simulink model "sistema_completo_discretizado_final"  (R2023b)
settings: Solver=FixedStepDiscrete  StartTime=0.0  StopTime=10.0  FixedStep=100e-6  RelTol=1e-3
values from neighbouring files (symbols this model uses):
  alpha_Cu = 3.9e-3    (= 0.0039)    [controlador_foc_simulink.m]    (also in parametros_planta.m; params_subsistema_termico.m; sistema_completo_en_codigo.m)
  beq_nom = bm + bl_nom/r^2    (= 2.19444444444e-05)    [parametros_planta.m]    (also in params_subsistema_mecanico.m; sistema_completo_en_codigo.m)
  Cts = 0.818    [parametros_planta.m]    (also in params_subsistema_termico.m)
  Jeq_nom = Jm + Jl_nom/r^2    (= 1.97847222222e-05)    [params_subsistema_mecanico.m]    (also in sistema_completo_en_codigo.m)
  kg_eq_nom = g*kl_nom/r    (= 0.0204305208333)    [params_subsistema_mecanico.m]    (also in sistema_completo_en_codigo.m)
  L_d = 6.6e-3    (= 0.0066)    [controlador_foc_simulink.m]    (also in params_subsistema_electromagnetico.m; sistema_completo_en_codigo.m)
  L_l = 0.8e-3    (= 0.0008)    [controlador_foc_simulink.m]    (also in params_subsistema_electromagnetico.m; sistema_completo_en_codigo.m)
  L_q = 5.8e-3    (= 0.0058)    [controlador_foc_simulink.m]    (also in params_subsistema_electromagnetico.m; sistema_completo_en_codigo.m)
  lambda_m = 0.016    [controlador_foc_simulink.m]    (also in parametros_planta.m; params_subsistema_electromagnetico.m; sistema_completo_en_codigo.m)
  Pp = 3    [controlador_foc_simulink.m]    (also in parametros_planta.m; params_subsistema_electromagnetico.m; sistema_completo_en_codigo.m)
  r = 120.0    (= 120)    [controlador_foc_simulink.m]    (also in parametros_planta.m; params_subsistema_mecanico.m; sistema_completo_en_codigo.m)
  Rs_REF = 1.02    [controlador_foc_simulink.m]    (also in parametros_planta.m; params_subsistema_termico.m; sistema_completo_en_codigo.m)
  Rts_amb = 146.7    [parametros_planta.m]    (also in params_subsistema_termico.m)
  Tamb = Tamb_max    (= 40)    [parametros_planta.m]    (also in params_subsistema_termico.m; sistema_completo_en_codigo.m)
  Ts_REF = 20.0    (= 20)    [controlador_foc_simulink.m]    (also in parametros_planta.m; params_subsistema_termico.m; sistema_completo_en_codigo.m)
undefined symbols (not defined in the file or in its folder): gain_i_1, gain_i_2, gain_pos_1, gain_pos_2, gain_T, K_v_amort, K_v_wn2, V_sat_max, V_sat_min, X0_ia, X0_ib, X0_ic, X0_pos, X0_T, X0_va, X0_vb, X0_vc
settings Model: Creator=Pc  LastModifiedBy=Gabriel

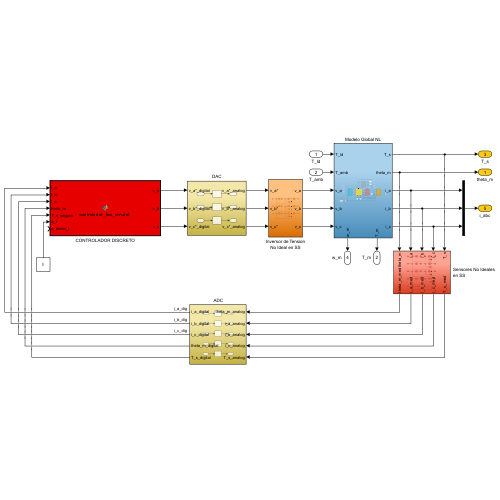
[thumbnail: Simulink's stored preview of the top-level diagram]
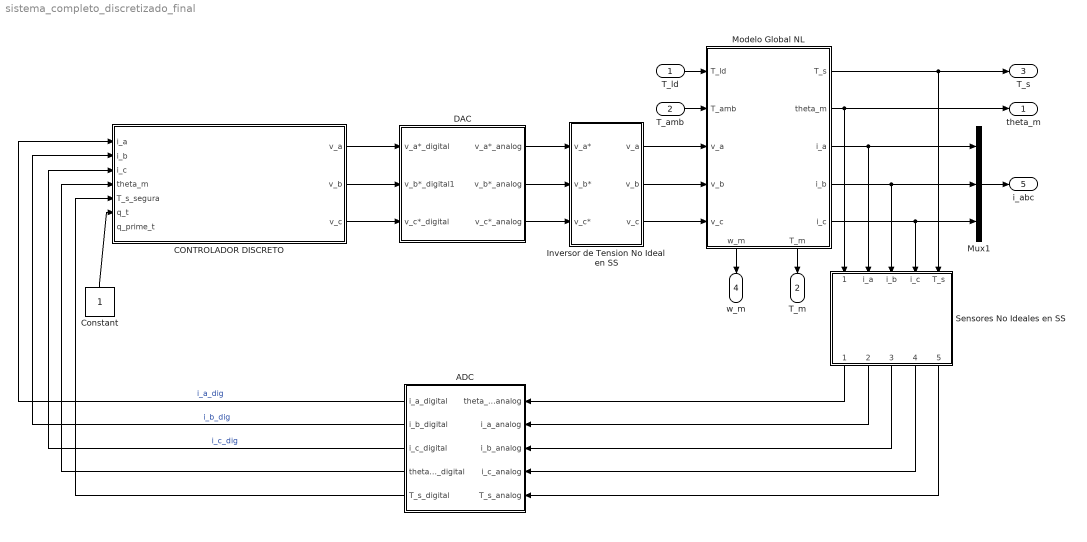
== system sistema_completo_discretizado_final ==
  T_ld : Inport
  T_amb : Inport  Port=2
  " ADC" : Subsystem
  CONTROLADOR DISCRETO : MATLAB Function  TreatAsAtomicUnit=on
  Constant : Constant
  DAC : Subsystem
  Inversor de Tension No Ideal en SS : Subsystem
  Modelo Global NL : Subsystem
      settings: PortSchema="{\"entries\":[{\"content\":{\"sides\":[{\"content\":{\"connectorIds\":[\"In1\",\"In2\",\"In3\",\"In4\",\"In5\"]},\"type\":\"ConnectorPlacement.EquallySpacedRectSide\",\"uuid\":\"386252be-5f39-4928-a151-52e681895a84\"},{\"content\":{\"connectorIds\":[\"Out1\",\"Out2\",\"Out3\",\"Out4\",\"Out5\"],\"side\":\"RIGHT\"},\"type\":\"ConnectorPlacement.EquallySpacedRectSide\",\"uuid\":\"aee83b90-e95b-4477-b157-a5534e7c5e6c\"},{\"content\":{\"side\":\"TOP\"},\"type\":\"ConnectorPlacement.EquallySpacedRectSide\",\"uuid\":\"e739b3f7-cae1-4498-b396-d13f7405e232\"},{\"content\":{\"connectorIds\":[\"Out6\",\"Out7\"],\"side\":\"BOTTOM\"},\"type\":\"ConnectorPlacement.EquallySpacedRectSide\",\"uuid\":\"86304fed-22cd-46a2-87e5-e7bae1c5cedf\"}]},\"type\":\"ConnectorPlacement.EquallySpacedConnector\",\"uuid\":\"c0eb110b-b212-4702-a1d5-9ec3ac2ff196\"}],\"packageUris\":[\"http://schema.mathworks.com/mf0/Connector/R2020b\"],\"version\":\"1.0\"}"
  Mux1 : Mux  Inputs=3
  Sensores No Ideales en SS : Subsystem
  theta_m : Outport
  T_m : Outport  Port=2
  T_s : Outport  Port=3
  w_m : Outport  Port=4
  i_abc : Outport  Port=5
  wires:
  Modelo Global NL/4(i_b) -> Sensores No Ideales en SS/3(i_b), Mux1/2
  T_amb/1 -> Modelo Global NL/2(T_amb)
  Sensores No Ideales en SS/5(T_s_med) -> " ADC"/5(T_s_analog)
  T_ld/1 -> Modelo Global NL/1(T_ld)
  Sensores No Ideales en SS/4(i_c_med) -> " ADC"/4(i_c_analog)
  Modelo Global NL/2(theta_m) -> Sensores No Ideales en SS/1(theta_m), theta_m/1
  Inversor de Tension No Ideal en SS/3(v_c) -> Modelo Global NL/5(v_c)
  Inversor de Tension No Ideal en SS/1(v_a) -> Modelo Global NL/3(v_a)
  Sensores No Ideales en SS/2(i_a_med) -> " ADC"/2(i_a_analog)
  Modelo Global NL/3(i_a) -> Sensores No Ideales en SS/2(i_a), Mux1/1
  Inversor de Tension No Ideal en SS/2(v_b) -> Modelo Global NL/4(v_b)
  Mux1/1 -> i_abc/1
  Modelo Global NL/1(T_s) -> Sensores No Ideales en SS/5(T_s), T_s/1
  Sensores No Ideales en SS/3(i_b_med) -> " ADC"/3(i_b_analog)
  Modelo Global NL/7(T_m) -> T_m/1
  DAC/2(v_b*_analog) -> Inversor de Tension No Ideal en SS/2(v_b*)
  DAC/3(v_c*_analog) -> Inversor de Tension No Ideal en SS/3(v_c*)
  Modelo Global NL/5(i_c) -> Sensores No Ideales en SS/4(i_c), Mux1/3
  Sensores No Ideales en SS/1(theta_m_med) -> " ADC"/1(theta_m_analog)
  Modelo Global NL/6(w_m) -> w_m/1
  DAC/1(v_a*_analog) -> Inversor de Tension No Ideal en SS/1(v_a*)
  CONTROLADOR DISCRETO/1(v_a) -> DAC/1(v_a*_digital)
  CONTROLADOR DISCRETO/2(v_b) -> DAC/2(v_b*_digital1)
  CONTROLADOR DISCRETO/3(v_c) -> DAC/3(v_c*_digital)
  " ADC"/1(i_a_digital) -> CONTROLADOR DISCRETO/1(i_a)  "i_a_dig"
  " ADC"/2(i_b_digital) -> CONTROLADOR DISCRETO/2(i_b)  "i_b_dig"
  " ADC"/3(i_c_digital) -> CONTROLADOR DISCRETO/3(i_c)  "i_c_dig"
  " ADC"/4(theta_m_digital) -> CONTROLADOR DISCRETO/4(theta_m)
  " ADC"/5(T_s_digital) -> CONTROLADOR DISCRETO/5(T_s_segura)
  Constant/1 -> CONTROLADOR DISCRETO/6(q_t)

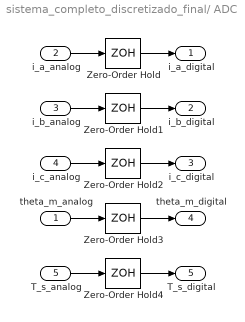
== system sistema_completo_discretizado_final/ ADC ==
  theta_m_analog : Inport
  i_a_analog : Inport  Port=2
  i_b_analog : Inport  Port=3
  i_c_analog : Inport  Port=4
  T_s_analog : Inport  Port=5
  Zero-Order Hold{,1..4} (5 alike) : ZeroOrderHold  SampleTime=100e-6
  i_a_digital : Outport
  i_b_digital : Outport  Port=2
  i_c_digital : Outport  Port=3
  theta_m_digital : Outport  Port=4
  T_s_digital : Outport  Port=5
  wires:
  theta_m_analog/1 -> Zero-Order Hold3/1
  i_a_analog/1 -> Zero-Order Hold/1
  Zero-Order Hold/1 -> i_a_digital/1
  i_c_analog/1 -> Zero-Order Hold2/1
  i_b_analog/1 -> Zero-Order Hold1/1
  T_s_analog/1 -> Zero-Order Hold4/1
  Zero-Order Hold1/1 -> i_b_digital/1
  Zero-Order Hold2/1 -> i_c_digital/1
  Zero-Order Hold3/1 -> theta_m_digital/1
  Zero-Order Hold4/1 -> T_s_digital/1

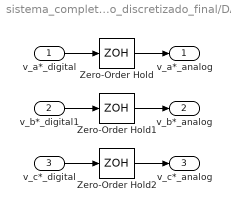
== system sistema_completo_discretizado_final/DAC ==
  v_a*_digital : Inport
  v_b*_digital1 : Inport  Port=2
  v_c*_digital : Inport  Port=3
  Zero-Order Hold : ZeroOrderHold  SampleTime=100e-6
  Zero-Order Hold1 : ZeroOrderHold  SampleTime=100e-6
  Zero-Order Hold2 : ZeroOrderHold  SampleTime=100e-6
  v_a*_analog : Outport
  v_b*_analog : Outport  Port=2
  v_c*_analog : Outport  Port=3
  wires:
  v_c*_digital/1 -> Zero-Order Hold2/1
  v_b*_digital1/1 -> Zero-Order Hold1/1
  v_a*_digital/1 -> Zero-Order Hold/1
  Zero-Order Hold/1 -> v_a*_analog/1
  Zero-Order Hold1/1 -> v_b*_analog/1
  Zero-Order Hold2/1 -> v_c*_analog/1

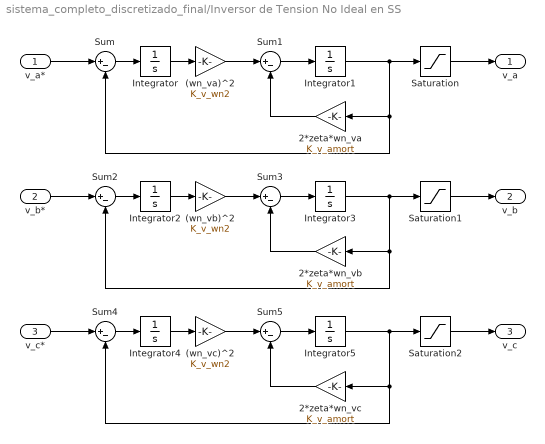
== system sistema_completo_discretizado_final/Inversor de Tension No Ideal en SS ==
  v_a* : Inport
  v_b* : Inport  Port=2
  v_c* : Inport  Port=3
  (wn_va)^2 : Gain  Gain=K_v_wn2
  (wn_vb)^2 : Gain  Gain=K_v_wn2
  (wn_vc)^2 : Gain  Gain=K_v_wn2
  2*zeta*wn_va : Gain  Gain=K_v_amort
  2*zeta*wn_vb : Gain  Gain=K_v_amort
  2*zeta*wn_vc : Gain  Gain=K_v_amort
  Integrator : Integrator  InitialCondition=X0_va(1)
  Integrator1 : Integrator  InitialCondition=X0_va(2)
  Integrator2 : Integrator  InitialCondition=X0_vb(1)
  Integrator3 : Integrator  InitialCondition=X0_vb(2)
  Integrator4 : Integrator  InitialCondition=X0_vc(1)
  Integrator5 : Integrator  InitialCondition=X0_vc(2)
  Saturation : Saturate  UpperLimit=V_sat_max  LowerLimit=V_sat_min
  Saturation1 : Saturate  UpperLimit=V_sat_max  LowerLimit=V_sat_min
  Saturation2 : Saturate  UpperLimit=V_sat_max  LowerLimit=V_sat_min
  Sum{,1..5} (6 alike) : Sum  Inputs=|+-
  v_a : Outport
  v_b : Outport  Port=2
  v_c : Outport  Port=3
  wires:
  Saturation1/1 -> v_b/1
  Saturation/1 -> v_a/1
  Saturation2/1 -> v_c/1
  Sum/1 -> Integrator/1
  v_a*/1 -> Sum/1
  (wn_va)^2/1 -> Sum1/1
  2*zeta*wn_va/1 -> Sum1/2
  Sum1/1 -> Integrator1/1
  Integrator1/1 -> 2*zeta*wn_va/1, Sum/2, Saturation/1
  Integrator/1 -> (wn_va)^2/1
  Integrator2/1 -> (wn_vb)^2/1
  Integrator3/1 -> Saturation1/1, Sum2/2, 2*zeta*wn_vb/1
  Sum3/1 -> Integrator3/1
  2*zeta*wn_vb/1 -> Sum3/2
  (wn_vb)^2/1 -> Sum3/1
  Sum2/1 -> Integrator2/1
  v_b*/1 -> Sum2/1
  Sum4/1 -> Integrator4/1
  (wn_vc)^2/1 -> Sum5/1
  2*zeta*wn_vc/1 -> Sum5/2
  Sum5/1 -> Integrator5/1
  Integrator5/1 -> Saturation2/1, 2*zeta*wn_vc/1, Sum4/2
  Integrator4/1 -> (wn_vc)^2/1
  v_c*/1 -> Sum4/1

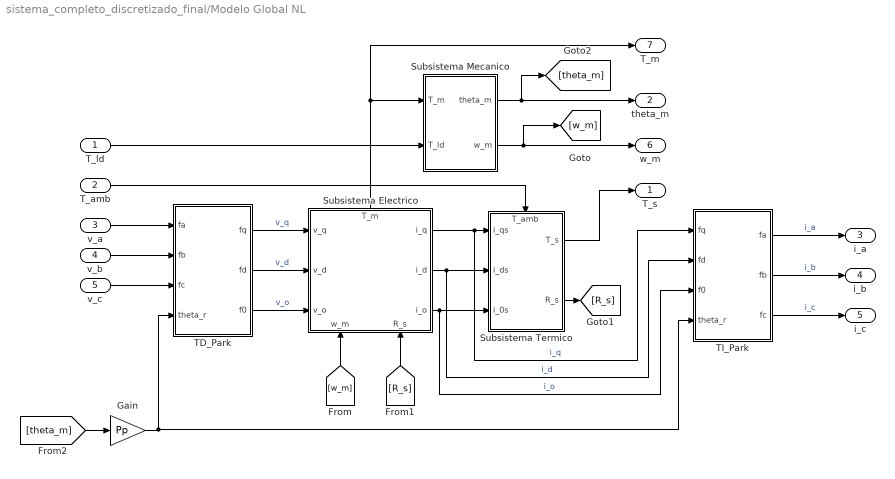
== system sistema_completo_discretizado_final/Modelo Global NL ==
  T_ld : Inport
  T_amb : Inport  Port=2
  v_a : Inport  Port=3
  v_b : Inport  Port=4
  v_c : Inport  Port=5
  Gain : Gain  Gain=Pp
  Subsistema Electrico : Subsystem
      settings: PortSchema="{\"entries\":[{\"content\":{\"sides\":[{\"content\":{\"connectorIds\":[\"In1\",\"In2\",\"In3\"]},\"type\":\"ConnectorPlacement.EquallySpacedRectSide\",\"uuid\":\"c7eb63ae-4015-4be9-a2f8-5ddbad38e871\"},{\"content\":{\"connectorIds\":[\"Out1\",\"Out2\",\"Out3\"],\"side\":\"RIGHT\"},\"type\":\"ConnectorPlacement.EquallySpacedRectSide\",\"uuid\":\"ed205027-9864-417a-9d2b-6eeb723ffec2\"},{\"content\":{\"connectorIds\":[\"Out4\"],\"side\":\"TOP\"},\"type\":\"ConnectorPlacement.EquallySpacedRectSide\",\"uuid\":\"5c5dee03-5728-4212-8fc2-a453d3484329\"},{\"content\":{\"connectorIds\":[\"In4\",\"In5\"],\"side\":\"BOTTOM\"},\"type\":\"ConnectorPlacement.EquallySpacedRectSide\",\"uuid\":\"494df340-b6d5-4f09-932e-9dbff39af1cf\"}]},\"type\":\"ConnectorPlacement.EquallySpacedConnector\",\"uuid\":\"0eeaea4c-3d80-4ebb-8c27-59b1b18764e9\"}],\"packageUris\":[\"http://schema.mathworks.com/mf0/Connector/R2020b\"],\"version\":\"1.0\"}"
  Subsistema Mecanico : Subsystem
  Subsistema Termico : Subsystem
      settings: PortSchema="{\"entries\":[{\"content\":{\"sides\":[{\"content\":{\"connectorIds\":[\"In1\",\"In2\",\"In3\"]},\"type\":\"ConnectorPlacement.EquallySpacedRectSide\",\"uuid\":\"5b1848a7-84bd-4673-a3fa-3976b4d0d5b9\"},{\"content\":{\"connectorIds\":[\"Out1\",\"Out2\"],\"side\":\"RIGHT\"},\"type\":\"ConnectorPlacement.EquallySpacedRectSide\",\"uuid\":\"feff3f8a-cd7c-43b1-91c3-7ab01b0b33a6\"},{\"content\":{\"connectorIds\":[\"In4\"],\"side\":\"TOP\"},\"type\":\"ConnectorPlacement.EquallySpacedRectSide\",\"uuid\":\"8de0b1b6-142f-442a-a92f-2baa615c6322\"}]},\"type\":\"ConnectorPlacement.EquallySpacedConnector\",\"uuid\":\"046fcb24-e0d9-4784-a784-7e36f9acbfbc\"}],\"packageUris\":[\"http://schema.mathworks.com/mf0/Connector/R2020b\"],\"version\":\"1.0\"}"
  TD_Park : MATLAB Function  TreatAsAtomicUnit=on
  TI_Park : MATLAB Function  TreatAsAtomicUnit=on
  T_s : Outport
  theta_m : Outport  Port=2
  i_a : Outport  Port=3
  i_b : Outport  Port=4
  i_c : Outport  Port=5
  w_m : Outport  Port=6
  T_m : Outport  Port=7
  wires:
  Subsistema Mecanico/1(theta_m) -> theta_m/1, [theta_m]
  TD_Park/2(fd) -> Subsistema Electrico/2(v_d)  "v_d"
  Subsistema Termico/1(T_s) -> T_s/1
  TD_Park/3(f0) -> Subsistema Electrico/3(v_o)  "v_o"
  Subsistema Mecanico/2(w_m) -> w_m/1, [w_m]
  [R_s] -> Subsistema Electrico/5(R_s)
  TI_Park/1(fa) -> i_a/1  "i_a"
  TD_Park/1(fq) -> Subsistema Electrico/1(v_q)  "v_q"
  Subsistema Electrico/4(T_m) -> T_m/1, Subsistema Mecanico/1(T_m)
  v_c/1 -> TD_Park/3(fc)
  Subsistema Electrico/2(i_d) -> Subsistema Termico/2(i_ds), TI_Park/2(fd)  "i_d"
  Subsistema Termico/2(R_s) -> [R_s]
  T_amb/1 -> Subsistema Termico/4(T_amb)
  T_ld/1 -> Subsistema Mecanico/2(T_ld)
  Subsistema Electrico/3(i_o) -> Subsistema Termico/3(i_0s), TI_Park/3(f0)  "i_o"
  TI_Park/2(fb) -> i_b/1  "i_b"
  Subsistema Electrico/1(i_q) -> TI_Park/1(fq), Subsistema Termico/1(i_qs)  "i_q"
  v_a/1 -> TD_Park/1(fa)
  v_b/1 -> TD_Park/2(fb)
  [w_m] -> Subsistema Electrico/4(w_m)
  TI_Park/3(fc) -> i_c/1  "i_c"
  [theta_m] -> Gain/1
  Gain/1 -> TD_Park/4(theta_r), TI_Park/4(theta_r)

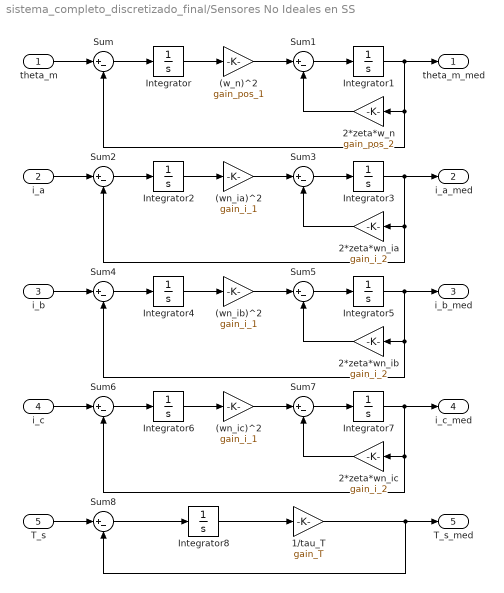
== system sistema_completo_discretizado_final/Sensores No Ideales en SS ==
  theta_m : Inport
  i_a : Inport  Port=2
  i_b : Inport  Port=3
  i_c : Inport  Port=4
  T_s : Inport  Port=5
  (w_n)^2 : Gain  Gain=gain_pos_1
  (wn_ia)^2 : Gain  Gain=gain_i_1
  (wn_ib)^2 : Gain  Gain=gain_i_1
  (wn_ic)^2 : Gain  Gain=gain_i_1
  1/tau_T : Gain  Gain=gain_T
  2*zeta*w_n : Gain  Gain=gain_pos_2
  2*zeta*wn_ia : Gain  Gain=gain_i_2
  2*zeta*wn_ib : Gain  Gain=gain_i_2
  2*zeta*wn_ic : Gain  Gain=gain_i_2
  Integrator : Integrator  InitialCondition=X0_pos(1)
  Integrator1 : Integrator  InitialCondition=X0_pos(2)
  Integrator2 : Integrator  InitialCondition=X0_ia(1)
  Integrator3 : Integrator  InitialCondition=X0_ia(2)
  Integrator4 : Integrator  InitialCondition=X0_ib(1)
  Integrator5 : Integrator  InitialCondition=X0_ib(2)
  Integrator6 : Integrator  InitialCondition=X0_ic(1)
  Integrator7 : Integrator  InitialCondition=X0_ic(2)
  Integrator8 : Integrator  InitialCondition=X0_T
  Sum{,1..8} (9 alike) : Sum  Inputs=|+-
  theta_m_med : Outport
  i_a_med : Outport  Port=2
  i_b_med : Outport  Port=3
  i_c_med : Outport  Port=4
  T_s_med : Outport  Port=5
  wires:
  i_a/1 -> Sum2/1
  theta_m/1 -> Sum/1
  Sum/1 -> Integrator/1
  Integrator/1 -> (w_n)^2/1
  (w_n)^2/1 -> Sum1/1
  2*zeta*w_n/1 -> Sum1/2
  Sum1/1 -> Integrator1/1
  Integrator1/1 -> theta_m_med/1, Sum/2, 2*zeta*w_n/1
  Integrator3/1 -> i_a_med/1, 2*zeta*wn_ia/1, Sum2/2
  Sum3/1 -> Integrator3/1
  2*zeta*wn_ia/1 -> Sum3/2
  (wn_ia)^2/1 -> Sum3/1
  Integrator2/1 -> (wn_ia)^2/1
  Sum2/1 -> Integrator2/1
  Sum4/1 -> Integrator4/1
  Integrator4/1 -> (wn_ib)^2/1
  (wn_ib)^2/1 -> Sum5/1
  2*zeta*wn_ib/1 -> Sum5/2
  Sum5/1 -> Integrator5/1
  Integrator5/1 -> i_b_med/1, Sum4/2, 2*zeta*wn_ib/1
  i_b/1 -> Sum4/1
  Integrator7/1 -> i_c_med/1, 2*zeta*wn_ic/1, Sum6/2
  Sum7/1 -> Integrator7/1
  2*zeta*wn_ic/1 -> Sum7/2
  (wn_ic)^2/1 -> Sum7/1
  Integrator6/1 -> (wn_ic)^2/1
  Sum6/1 -> Integrator6/1
  i_c/1 -> Sum6/1
  Sum8/1 -> Integrator8/1
  Integrator8/1 -> 1/tau_T/1
  T_s/1 -> Sum8/1
  1/tau_T/1 -> Sum8/2, T_s_med/1

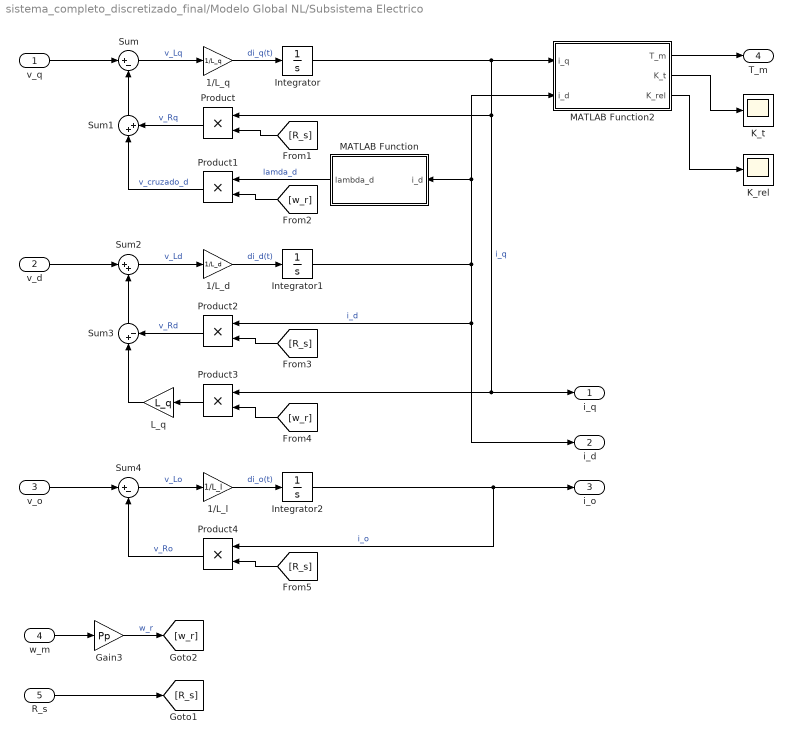
== system sistema_completo_discretizado_final/Modelo Global NL/Subsistema Electrico ==
  v_q : Inport
  v_d : Inport  Port=2
  v_o : Inport  Port=3
  w_m : Inport  Port=4
  R_s : Inport  Port=5
  1/L_d : Gain  Gain=1/L_d
  1/L_l : Gain  Gain=1/L_l
  1/L_q : Gain  Gain=1/L_q
  Gain3 : Gain  Gain=Pp
  Integrator : Integrator
  Integrator1 : Integrator
  Integrator2 : Integrator
  K_rel : Scope
  K_t : Scope
  L_q : Gain  Gain=L_q
  MATLAB Function : MATLAB Function  TreatAsAtomicUnit=on
  MATLAB Function2 : MATLAB Function  TreatAsAtomicUnit=on
  Product{,1..4} (5 alike) : Product
  Sum : Sum  Inputs=|+-
  Sum1 : Sum  Inputs=|++
  Sum2 : Sum  Inputs=|++
  Sum3 : Sum  Inputs=|+-
  Sum4 : Sum  Inputs=|+-
  i_q : Outport
  i_d : Outport  Port=2
  i_o : Outport  Port=3
  T_m : Outport  Port=4
  wires:
  Integrator/1 -> MATLAB Function2/1(i_q), Product/1, i_q/1, Product3/1  "i_q"
  Sum3/1 -> Sum2/2
  Product1/1 -> Sum1/1  "v_cruzado_d"
  Integrator1/1 -> MATLAB Function2/2(i_d), MATLAB Function/1(i_d), i_d/1, Product2/1  "i_d"
  Sum1/1 -> Sum/2
  1/L_d/1 -> Integrator1/1  "di_d(t)"
  MATLAB Function/1(lambda_d) -> Product1/1  "lamda_d"
  Sum4/1 -> 1/L_l/1  "v_Lo"
  [w_r] -> Product3/2
  Sum/1 -> 1/L_q/1  "v_Lq"
  1/L_l/1 -> Integrator2/1  "di_o(t)"
  Integrator2/1 -> i_o/1, Product4/1  "i_o"
  Product2/1 -> Sum3/2  "v_Rd"
  Product/1 -> Sum1/2  "v_Rq"
  [R_s] -> Product4/2
  Product3/1 -> L_q/1
  1/L_q/1 -> Integrator/1  "di_q(t)"
  Sum2/1 -> 1/L_d/1  "v_Ld"
  v_q/1 -> Sum/1
  [R_s] -> Product/2
  Product4/1 -> Sum4/2  "v_Ro"
  [w_r] -> Product1/2
  [R_s] -> Product2/2
  L_q/1 -> Sum3/1
  v_d/1 -> Sum2/1
  v_o/1 -> Sum4/1
  MATLAB Function2/1(T_m) -> T_m/1
  MATLAB Function2/3(K_rel) -> K_rel/1
  MATLAB Function2/2(K_t) -> K_t/1
  w_m/1 -> Gain3/1
  R_s/1 -> [R_s]
  Gain3/1 -> [w_r]  "w_r"

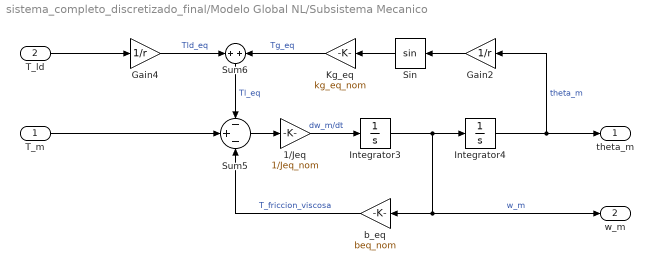
== system sistema_completo_discretizado_final/Modelo Global NL/Subsistema Mecanico ==
  T_m : Inport
  T_ld : Inport  Port=2
  1/Jeq : Gain  Gain=1/Jeq_nom
  Gain2 : Gain  Gain=1/r
  Gain4 : Gain  Gain=1/r
  Integrator3 : Integrator
  Integrator4 : Integrator
  Kg_eq : Gain  Gain=kg_eq_nom
  Sin : Trigonometry
  Sum5 : Sum  Inputs=-+-
  Sum6 : Sum  Inputs=+|+
  b_eq : Gain  Gain=beq_nom
  theta_m : Outport
  w_m : Outport  Port=2
  wires:
  Sin/1 -> Kg_eq/1
  Gain4/1 -> Sum6/1  "Tld_eq"
  Integrator4/1 -> theta_m/1, Gain2/1  "theta_m"
  Kg_eq/1 -> Sum6/2  "Tg_eq"
  Sum5/1 -> 1/Jeq/1
  b_eq/1 -> Sum5/3  "T_friccion_viscosa"
  T_m/1 -> Sum5/2
  Gain2/1 -> Sin/1
  Sum6/1 -> Sum5/1  "Tl_eq"
  Integrator3/1 -> w_m/1, b_eq/1, Integrator4/1  "w_m"
  T_ld/1 -> Gain4/1
  1/Jeq/1 -> Integrator3/1  "dw_m/dt"

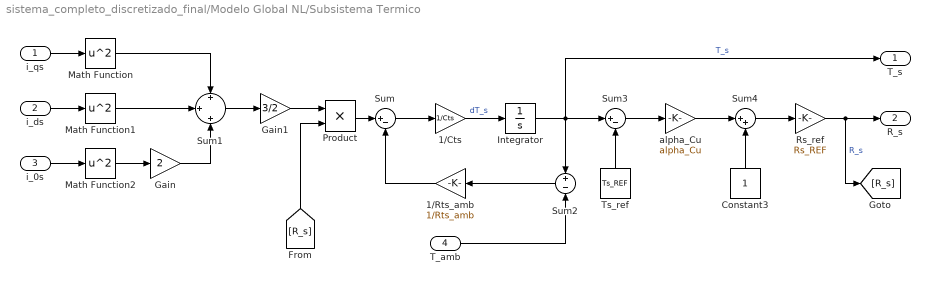
== system sistema_completo_discretizado_final/Modelo Global NL/Subsistema Termico ==
  i_qs : Inport
  i_ds : Inport  Port=2
  i_0s : Inport  Port=3
  T_amb : Inport  Port=4
  1/Cts : Gain  Gain=1/Cts
  1/Rts_amb : Gain  Gain=1/Rts_amb
  Constant3 : Constant
  Gain : Gain  Gain=2
  Gain1 : Gain  Gain=3/2
  Integrator : Integrator  InitialCondition=Tamb
  Math Function : Math  Operator=square
  Math Function1 : Math  Operator=square
  Math Function2 : Math  Operator=square
  Product : Product
  Rs_ref : Gain  Gain=Rs_REF
  Sum : Sum  Inputs=|+-
  Sum1 : Sum  Inputs=+|+|+
  Sum2 : Sum  Inputs=+-
  Sum3 : Sum  Inputs=|+-
  Sum4 : Sum  Inputs=|++
  Ts_ref : Constant  Value=Ts_REF
  alpha_Cu : Gain  Gain=alpha_Cu
  T_s : Outport
  R_s : Outport  Port=2
  wires:
  1/Cts/1 -> Integrator/1  "dT_s"
  Sum3/1 -> alpha_Cu/1
  Rs_ref/1 -> R_s/1, [R_s]  "R_s"
  Sum4/1 -> Rs_ref/1
  [R_s] -> Product/2
  i_ds/1 -> Math Function1/1
  Constant3/1 -> Sum4/2
  Integrator/1 -> T_s/1, Sum2/1, Sum3/1  "T_s"
  Math Function1/1 -> Sum1/2
  alpha_Cu/1 -> Sum4/1
  Sum2/1 -> 1/Rts_amb/1
  Product/1 -> Sum/1
  i_qs/1 -> Math Function/1
  Sum/1 -> 1/Cts/1
  T_amb/1 -> Sum2/2
  Math Function/1 -> Sum1/1
  i_0s/1 -> Math Function2/1
  1/Rts_amb/1 -> Sum/2
  Ts_ref/1 -> Sum3/2
  Math Function2/1 -> Gain/1
  Gain/1 -> Sum1/3
  Sum1/1 -> Gain1/1
  Gain1/1 -> Product/1

== matlab function sistema_completo_discretizado_final/Modelo Global NL/TD_Park ==
  data: fa input; fq output; fb input; fc input; theta_r input; fd output; f0 output
function [fq, fd, f0] = T_Park(fa, fb, fc, theta_r)
%#codegen
% Transformada directa de Park: abc -> qd0
% Convención usada:
% fq: eje q
% fd: eje d
% f0: componente homopolar

c1 = cos(theta_r);
c2 = cos(theta_r - 2*pi/3);
c3 = cos(theta_r + 2*pi/3);

s1 = sin(theta_r);
s2 = sin(theta_r - 2*pi/3);
s3 = sin(theta_r + 2*pi/3);

fq = (2/3)*(c1*fa + c2*fb + c3*fc);
fd = (2/3)*(s1*fa + s2*fb + s3*fc);
f0 = (1/3)*(fa + fb + fc);
end

== matlab function sistema_completo_discretizado_final/Modelo Global NL/Subsistema Electrico/MATLAB Function ==
  data: i_d input; lambda_d output; lambda_m parameter; L_d parameter
function lambda_d = calcular_flujo_d(i_d, lambda_m, L_d)
    % CALCULAR_FLUJO_D Calcula el flujo magnético total concatenado en el eje directo (d).
    %
    % Entradas:
    %   i_d      : Corriente instantánea en el eje d (Señal dinámica de entrada).
    %   lambda_m : Flujo de los imanes permanentes (Parámetro estático).
    %   L_d      : Inductancia del estator en el eje d (Parámetro estático).
    %
    % Salida:
    %   lambda_d : Flujo magnético total en el eje d.

    % Cálculo: Flujo de imanes + Flujo de reacción del inducido
    lambda_d = lambda_m + L_d * i_d;
end

== matlab function sistema_completo_discretizado_final/Modelo Global NL/Subsistema Electrico/MATLAB Function2 ==
  data: i_q input; i_d input; T_m output; Pp parameter; lambda_m parameter; L_d parameter; L_q parameter; K_t output; K_rel output
function [T_m, K_t, K_rel] = calcular_torque(i_q, i_d, Pp, lambda_m, L_d, L_q)
    % CALCULAR_TORQUE Calcula el torque electromagnético total de la máquina PMSM
    % y sus constantes equivalentes.
    % 
    % Entradas dinámicas (Inports):
    %   i_q      : Corriente en el eje en cuadratura [A].
    %   i_d      : Corriente en el eje directo [A].
    %
    % Parámetros estáticos (Parameters):
    %   P_p      : Número de pares de polos.
    %   lambda_m : Flujo magnético de los imanes permanentes [Wb].
    %   L_d      : Inductancia del eje d [H].
    %   L_q      : Inductancia del eje q [H].
    %
    % Salidas:
    %   T_m      : Torque electromagnético generado [N.m].
    %   K_t      : Constante de torque de alineación [N.m/A].
    %   K_rel    : Constante de torque de reluctancia [N.m/A^2].

    % 1. Cálculo de las constantes 
    K_t = (3/2) * Pp * lambda_m;
    K_rel = (3/2) * Pp * (L_d - L_q);

    % 2. Cálculo del torque electromagnético total
    T_m = K_t * i_q + K_rel * i_d * i_q;
end

== matlab function sistema_completo_discretizado_final/Modelo Global NL/TI_Park ==
  data: fq input; fa output; fd input; f0 input; theta_r input; fb output; fc output
function [fa, fb, fc] = TI_Park(fq, fd, f0, theta_r)
%#codegen
% Transformada inversa de Park: qd0 -> abc

fa = cos(theta_r)*fq ...
   + sin(theta_r)*fd ...
   + f0;

fb = cos(theta_r - 2*pi/3)*fq ...
   + sin(theta_r - 2*pi/3)*fd ...
   + f0;

fc = cos(theta_r + 2*pi/3)*fq ...
   + sin(theta_r + 2*pi/3)*fd ...
   + f0;
end

== matlab function sistema_completo_discretizado_final/CONTROLADOR DISCRETO ==
  settings: updateMethod=DISCRETE  sampleTime=100e-6
  data: i_a input; v_a output; i_b input; i_c input; theta_m input; T_s_segura input; q_t input; q_prime_t input; v_b output; v_c output
function [v_a, v_b, v_c] = controlador_foc_simulink(i_a, i_b, i_c, theta_m, T_s_segura, q_t, q_prime_t)


    %% SECCIÓN 1: CONFIGURACION Y VAR. GLOBALES (#define y variables globales)
    % En la generación de código C, el compilador tratará todo esto como constantes.

    % ===== PARAMETRO DE MUESTREO =====
    T_s = 100e-6;   % [s] 10 KHz
    
    % ===== SUBSISTEMA MECANICO =====
    g = 9.80665;    % [m/s^2] Aceleración de la gravedad
    r = 120.0;      % [-] Relación de reducción total
    
    bl_nom = 0.10;          % [N*m/(rad/s)]
    m   = 1.0;       % [kg] Masa del brazo
    Lcm = 0.25;      % [m] Distancia del centro de masa a la articulación
    Jcm = 0.0208;    % [kg*m^2] Inercia respecto del centro de masa
    Ll  = 0.50;      % [m] Longitud hasta el extremo
    ml_nom = 0.0;    % [kg]

    Jm = 14.0e-6;    % [kg*m^2]
    bm = 15.0e-6;    % [N*m/(rad/s)]

    Jl_nom = (m*Lcm^2 + Jcm) + ml_nom*Ll^2;
    kl_nom = m*Lcm + ml_nom*Ll;
    
    Jeq_ctrl   = Jm + Jl_nom/r^2;
    beq_ctrl   = bm + bl_nom/r^2;
    kg_eq_ctrl = g*kl_nom/r;
    Jeq_obs    = Jeq_ctrl;
    beq_obs    = beq_ctrl;
    
    % ===== SUBSISTEMA ELECTRICO =====
    Pp       = 3;          % [-] Pares de polos
    lambda_m = 0.016;      % [Wb] Flujo concatenado de los imanes
    L_q      = 5.8e-3;     % [H] Inductancia del eje q
    L_d      = 6.6e-3;     % [H] Inductancia del eje d
    L_l      = 0.8e-3;     % [H] Inductancia de dispersión / eje cero
    
    K_t   = (3/2)*Pp*lambda_m;       % [N*m/A] Constante de torque con i_d = 0
    K_rel = (3/2)*Pp*(L_d - L_q);    % [N*m/A^2] Componente de reluctancia
    
    % ===== SUBSISTEMA TÉRMICO =====
    Rs_REF   = 1.02;     % [ohm/fase] A Ts_REF
    Ts_REF   = 20.0;     % [°C]
    alpha_Cu = 3.9e-3;   % [1/°C]
    
    % ===== GANANCIAS OBSERVADOR DE ESTADO =====
    polo_obs_deseado = -3200;    % [rad/s] Dos polos coincidentes
    K_eth_num = 3 * abs(polo_obs_deseado);
    K_ew_num  = 3 * abs(polo_obs_deseado)^2;
    K_ei_num  = abs(polo_obs_deseado)^3;
    
    % ===== GANANCIAS CONTROLADORES =====
    p_c = -5000;                 % [rad/s] Polo deseado de los lazos de corriente
    R_q_num = -p_c*L_q;          % [ohm]
    R_d_num = -p_c*L_d;          % [ohm]
    R_o_num = -p_c*L_l;          % [ohm]
    
    wn_pid   = 800;              % [rad/s]
    zeta_pid = 0.75;             % [-]
    n_pid    = 2*zeta_pid + 1;   % n = 2.5
    
    ba_num   = Jeq_ctrl*n_pid*wn_pid;
    Ksa_num  = Jeq_ctrl*n_pid*wn_pid^2;
    Ksia_num = Jeq_ctrl*wn_pid^3;
    Torque_max = 45;

    %% SECCIÓN 2: INICIALIZACIÓN DE MEMORIA (ESTADOS)
    persistent T_m_star_prev
    
    if isempty(T_m_star_prev)
        T_m_star_prev = 0;
    end
    
    % Consignas fijas para control FOC estándar
    i_d_star = 0; 
    i_o_star = 0;
    
    %% SECCIÓN 3: EJECUCIÓN DEL LAZO (Simula 1 ciclo del Timer)
    % Se ejecutara una vez cada T_s segundos

    % 1. Preparacion 
    theta_r = calcular_theta_r(theta_m);
    R_s = estimar_Rs(T_s_segura);
        
    % Transformacion de Park (abc -> qd0)
    [i_q, i_d, i_o] = T_Park(i_a, i_b, i_c, theta_r);
        
    % Observador de Estado (Usando el T_m_star del ciclo anterior)
    [w_m_estimada, theta_m_estimada] = observador_estado(theta_m, T_m_star_prev);
        
    % Lazo Externo (Velocidad / Posición)
    [theta_m_star, w_m_star] = set_point_discreto(q_t, q_prime_t);

    T_m_star = controlador_pid(w_m_star, w_m_estimada);
        
    % Lazo Interno (Corriente)
    i_q_star = compensador_mecanico(T_m_star, w_m_estimada, theta_m, i_d);

    [v_q, v_d, v_o] = controlador_corriente(i_q_star, i_d_star, i_o_star, i_q, i_d, i_o, R_s, w_m_estimada);
                                                
    % Transformacion Inversa de Park (qd0 -> abc)
    [v_a, v_b, v_c] = TI_Park(v_q, v_d, v_o, theta_r);
        
    % Actualizar la Memoria para proximo ciclo
    T_m_star_prev = T_m_star; 
    
    %% SECCIÓN 4: MODULOS DE CONTROL
    % Funciones que toman mediciones o calculan referencias
    
    function [theta_m_star, w_m_star] = set_point_discreto(q_t, q_prime_t)
        % Definición de variables de memoria (persistent)
        persistent q_t_prev q_prime_prev theta_int_prev
    
        % Inicialización en el primer ciclo de ejecución (t=0)
        if isempty(q_t_prev)
            q_t_prev = q_t;             % Evita el pico (infinito) de la derivada en t=0
            q_prime_prev = q_prime_t;
            theta_int_prev = 0;         % El integrador arranca descargado
        end
    
        % --- CÁLCULO NUMÉRICO DISCRETO ---
        % A. Derivador Discreto (Diferencia Hacia Atrás / Backward Euler)
        q_dot_derivado = (q_t - q_t_prev) / T_s;
    
        % B. Integrador Discreto (Método de Tustin / Trapezoidal)
        theta_integrado = theta_int_prev + (T_s / 2) * (q_prime_t + q_prime_prev);
    
        % --- SALIDAS DEL SISTEMA ---
        theta_m_star = r * (q_t + theta_integrado);
        w_m_star     = r * (q_prime_t + q_dot_derivado);
    
        % Actualización de memoria para el próximo ciclo
        q_t_prev = q_t;
        q_prime_prev = q_prime_t;
        theta_int_prev = theta_integrado;
    end
    
    function T_m_star = controlador_pid(w_m_star, w_m)
        % Memoria de estados para los integradores y valores previos
        persistent e_pos_estado e_int_estado e_vel_prev e_pos_prev
        
        % Inicialización en el primer ciclo (t=0)
        if isempty(e_pos_estado)
            e_pos_estado = 0; % Memoria del integrador de posición
            e_int_estado = 0; % Memoria del integrador de la acción integral
            e_vel_prev = 0;   % Velocidad del ciclo anterior
            e_pos_prev = 0;   % Posición del ciclo anterior
        end
    
        % Cálculo del Error de Velocidad
        e_vel = w_m_star - w_m;
    
        % Primer Integrador: Error de Velocidad -> Error de Posición
        e_pos = e_pos_estado + (T_s / 2) * (e_vel + e_vel_prev);
        
        % Segundo Integrador: Error de Posición -> Integral del error de posición
        e_int = e_int_estado + (T_s / 2) * (e_pos + e_pos_prev);
        
        D_action = ba_num * e_vel;
        P_action = Ksa_num * e_pos;
        I_action = Ksia_num * e_int;
    
        % --- CALCULO DE LA SALIDA ---
        T_m_star_unbounded = P_action + I_action + D_action;
    
        % --- SATURACIÓN DE SALIDA ---
        if T_m_star_unbounded > Torque_max
            T_m_star = Torque_max;
            % Saturado: No guardamos el nuevo e_int en e_int_estado (congelamos el integrador I)
        elseif T_m_star_unbounded < -Torque_max
            T_m_star = -Torque_max;
            % Saturado: No guardamos el nuevo e_int en e_int_estado (congelamos el integrador I)
        else
            T_m_star = T_m_star_unbounded;
            % Zona lineal: Actualizamos la memoria del integrador I
            e_int_estado = e_int; 
        end
    
        % El integrador de posición NUNCA se congela, solo el de integracion.
        e_pos_estado = e_pos;
    
        % Actualización de memorias para el cálculo de Tustin en el próximo ciclo
        e_vel_prev = e_vel;
        e_pos_prev = e_pos;
    end
    
    function i_q_star = compensador_mecanico(T_m_star, w_m_estimada, theta_m, i_d)
        % Compensación Feedforward de Fricción Viscosa
        T_friccion = beq_ctrl * w_m_estimada;
    
        % Compensación Feedforward de Gravedad
        T_gravedad = kg_eq_ctrl * sin(theta_m / r);
    
        % Torque Total Requerido
        T_req = T_m_star + T_friccion + T_gravedad;
    
        % --- Modulación de Torque a Corriente ---
        % T = (K_t + K_rel * i_d) * i_q
        Denominador_Torque = K_t + K_rel * i_d;
    
        % Evitar división por cero
        if abs(Denominador_Torque) < 1e-6
            Denominador_Torque = sign(Denominador_Torque) * 1e-6;
            if Denominador_Torque == 0
                Denominador_Torque = 1e-6;
            end
        end
    
        % Cálculo final de la consigna de corriente
        i_q_star = T_req / Denominador_Torque;
    end
    
    function [v_q, v_d, v_o] = controlador_corriente(i_q_star, i_d_star, i_o_star, i_q, i_d, i_o, R_s, w_m_estimada)
        % --- Controlador Proporcional ---
        % Cálculo del error de seguimiento
        e_q = i_q_star - i_q;
        e_d = i_d_star - i_d;
        e_o = i_o_star - i_o;
        
        % Generación de las tensiones de control
        v_bar_q = R_q_num * e_q;
        v_bar_d = R_d_num * e_d;
        v_bar_o = R_o_num * e_o;
    
        % --- Desacoplamiento electrico (Feedback Linearization) ---
        % Eje en Cuadratura (q): Compensa caída óhmica y fuerza contraelectromotriz
        v_q = v_bar_q + R_s * i_q + Pp * w_m_estimada * (L_d * i_d + lambda_m);
        
        % Eje Directo (d): Compensa caída óhmica y acoplamiento por reluctancia cruzada
        v_d = v_bar_d + R_s * i_d - Pp * w_m_estimada * L_q * i_q;
        
        % Eje Homopolar (0): Compensa únicamente caída óhmica
        v_o = v_bar_o + R_s * i_o;
    end
    
    %% SECCIÓN 5: OBSERVADORES Y ESTIMADORES
    % Funciones que infieren el estado del sistema a partir de mediciones
    
    function [w_m_estimada, theta_m_estimada] = observador_estado(theta_m, T_m_star)
        % Memoria de los integradores (Salidas)
        persistent int1_estado w_est_estado th_est_estado
        
        % Memoria de las entradas a los integradores (para método de Tustin)
        persistent in1_prev in2_prev in3_prev
        
        % Inicialización
        if isempty(th_est_estado)
            int1_estado = 0;   
            w_est_estado = 0;    
            th_est_estado = 0;  
            
            in1_prev = 0;
            in2_prev = 0;
            in3_prev = 0;
        end
        
        % Cálculo del error de estimación (usando la posición estimada previa)
        e_theta = theta_m - th_est_estado;
        
        % --- Lazo de Perturbación (K_ei) ---
        in1_actual = K_ei_num * e_theta;
        int1_actual = int1_estado + (T_s / 2) * (in1_actual + in1_prev); % Salida del 1er integrador
        
        % --- Lazo de Velocidad (K_ew) ---
        in2_actual = (T_m_star / Jeq_obs) + int1_actual + (K_ew_num * e_theta);
        w_est_actual = w_est_estado + (T_s / 2) * (in2_actual + in2_prev); % Salida del 2do integrador
        
        % --- Lazo de Posición (K_eth) ---
        in3_actual = w_est_actual + (K_eth_num * e_theta);
        th_est_actual = th_est_estado + (T_s / 2) * (in3_actual + in3_prev); % Salida del 3er integrador
        
        % --- ASIGNACIÓN DE SALIDAS ---
        w_m_estimada = w_est_actual;
        theta_m_estimada = th_est_actual;
        
        % --- ACTUALIZACIÓN DE MEMORIAS PARA EL PRÓXIMO CICLO ---
        % Actualizamos los estados de los integradores
        int1_estado = int1_actual;
        w_est_estado = w_est_actual;
        th_est_estado = th_est_actual;
        
        % Actualizamos las entradas previas para el cálculo de Tustin
        in1_prev = in1_actual;
        in2_prev = in2_actual;
        in3_prev = in3_actual;
    end
    
    function R_s = estimar_Rs(T_s_segura)
        % Cálculo del incremento de temperatura
        Delta_T = T_s_segura - Ts_REF;
    
        % Aplicación de la Ecuación del modelo físico
        R_s = Rs_REF * (1 + alpha_Cu * Delta_T);
    end
    
    %% SECCIÓN 6: MATEMÁTICA Y TRANSFORAMACIONES (utils.c)
    % Funciones algebraicas, sin memoria ni estados
    
    function theta_r = calcular_theta_r(theta_m)
        theta_r = Pp * theta_m;
    end
    
    function [fq, fd, f0] = T_Park(fa, fb, fc, theta_r)
        % Transformada directa de Park: abc -> qd0
        c1 = cos(theta_r);
        c2 = cos(theta_r - 2*pi/3);
        c3 = cos(theta_r + 2*pi/3);
        
        s1 = sin(theta_r);
        s2 = sin(theta_r - 2*pi/3);
        s3 = sin(theta_r + 2*pi/3);
        
        fq = (2/3)*(c1*fa + c2*fb + c3*fc);
        fd = (2/3)*(s1*fa + s2*fb + s3*fc);
        f0 = (1/3)*(fa + fb + fc);
    end
    
    function [fa, fb, fc] = TI_Park(fq, fd, f0, theta_r)
        % Transformada inversa de Park: qd0 -> abc
        fa = cos(theta_r)*fq ...
           + sin(theta_r)*fd ...
           + f0;
        
        fb = cos(theta_r - 2*pi/3)*fq ...
           + sin(theta_r - 2*pi/3)*fd ...
           + f0;
        
        fc = cos(theta_r + 2*pi/3)*fq ...
           + sin(theta_r + 2*pi/3)*fd ...
           + f0;
    end
end
